simulink model "beta_estimators_simulink"  (R2017a)
settings: Solver=VariableStepAuto  StartTime=0.0  StopTime=10.0  FixedStep=1e-3  RelTol=1e-3
values from neighbouring files (symbols this model uses):
  Den_PDa = [1,(Na*Tsa-2)/(Na*Tsa+2)]    [rosbag_reader_simulink_GammaEstimators.m]
  FilterDTF = c2d(FilterCTF,Ts_filter,'tustin')    [rosbag_reader_simulink_GammaEstimators.m]
  Kp = 10*2*pi    (= 62.8318530718)    [rosbag_reader_simulink_GammaEstimators.m]    (also in taraPDscript.m = 628.318530718)
  Num_PDa = [(Kpa*(2+Na*Tsa)+2*Kda*Na)/(2+Na*Tsa),(-2*Kpa+Na*Tsa*Kpa-2*Kda*Na)/(2+Na*Tsa)]    [rosbag_reader_simulink_GammaEstimators.m]
  x0_acc = [X_opt.Data(1),Y_opt.Data(1),gamma_opt_spline.Data(1),V_opt.Data(1)]    [rosbag_reader_simulink_GammaEstimators.m]
  x0_vel = [X_opt.Data(1),Y_opt.Data(1),gamma_opt_spline.Data(1)]    [rosbag_reader_simulink_GammaEstimators.m]
undefined symbols (not defined in the file or in its folder): DiscIntNeverNeededParam
libraries: dspsigops x2
settings Model: Creator=bascetta  LastModifiedBy=marco
settings OptimizationCC: DefaultParameterBehavior=Inlined  PassReuseOutputArgsAs=Individual arguments  MaxStackSize=64
settings DebuggingCC: ParameterTunabilityLossMsg=error
settings HardwareCC: ProdBitPerPointer=32  ProdBitPerSizeT=32  ProdBitPerPtrDiffT=32  ProdLargestAtomicFloat=None  ProdIntDivRoundTo=Undefined  ProdEndianess=Unspecified  ProdWordSize=32  ProdHWDeviceType=Generic->Unspecified (assume 32-bit Generic)
settings SFSimCC: MATLABDynamicMemAlloc=off
settings RTWCC: SystemTargetFile=ert.tlc  TemplateMakefile=ert_default_tmf  Description=Embedded Coder  GenerateReport=on  Toolchain=Catkin  IncludeHyperlinkInReport=on  LaunchReport=on  GenerateTraceInfo=on  GenerateTraceReport=on  GenerateTraceReportSl=on  GenerateTraceReportSf=on  GenerateTraceReportEml=on
settings CodeAppCC: ForceParamTrailComments=on  IgnoreCustomStorageClasses=off  OperatorAnnotations=on  SimulinkDataObjDesc=on  SFDataObjDesc=on  MATLABFcnDesc=on  InsertBlockDesc=on  MATLABSourceComments=on
settings ERTTargetCC: ERTCustomFileTemplate=example_file_process.tlc

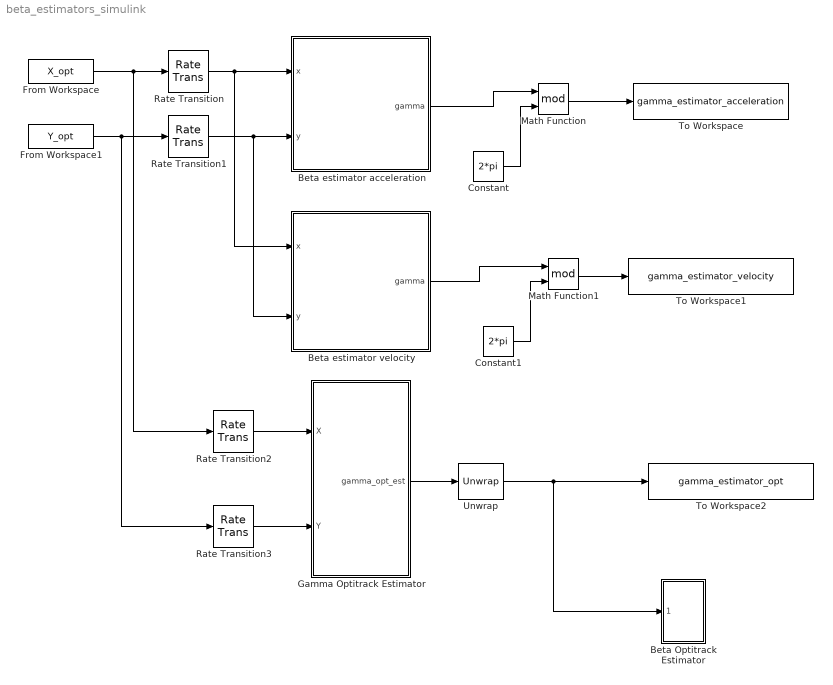
== system beta_estimators_simulink ==
  Beta Optitrack Estimator : Subsystem
  Beta estimator acceleration : Subsystem  TreatAsAtomicUnit=on  SystemSampleTime=1e-3
  Beta estimator velocity : Subsystem
  Constant : Constant  Value=2*pi
  Constant1 : Constant  Value=2*pi
  From Workspace : FromWorkspace  VariableName=X_opt  SampleTime=0  Interpolate=off  OutputAfterFinalValue=Holding final value
  From Workspace1 : FromWorkspace  VariableName=Y_opt  SampleTime=0  Interpolate=off  OutputAfterFinalValue=Holding final value
  Gamma Optitrack Estimator : Subsystem  TreatAsAtomicUnit=on  SystemSampleTime=0.01
  Math Function : Math  Operator=mod  OutputSignalType=real  SaturateOnIntegerOverflow=on
  Math Function1 : Math  Operator=mod  OutputSignalType=real  SaturateOnIntegerOverflow=on
  Rate Transition{,1..3} (4 alike) : RateTransition
  To Workspace : ToWorkspace  VariableName=gamma_estimator_acceleration  SaveFormat=Timeseries  SampleTime=-1
  To Workspace1 : ToWorkspace  VariableName=gamma_estimator_velocity  SaveFormat=Timeseries  SampleTime=-1
  To Workspace2 : ToWorkspace  VariableName=gamma_estimator_opt  SaveFormat=Timeseries  SampleTime=-1
  Unwrap : dspsigops/Unwrap  tol=pi  InputProcessing=Columns as channels (frame based)  running=off
  wires:
  From Workspace1/1 -> Rate Transition3/1, Rate Transition1/1
  Math Function/1 -> To Workspace/1
  Constant/1 -> Math Function/2
  Beta estimator acceleration/1(gamma) -> Math Function/1
  From Workspace/1 -> Rate Transition2/1, Rate Transition/1
  Math Function1/1 -> To Workspace1/1
  Constant1/1 -> Math Function1/2
  Beta estimator velocity/1(gamma) -> Math Function1/1
  Rate Transition/1 -> Beta estimator velocity/1(x), Beta estimator acceleration/1(x)
  Rate Transition1/1 -> Beta estimator velocity/2(y), Beta estimator acceleration/2(y)
  Rate Transition2/1 -> Gamma Optitrack Estimator/1(X)
  Rate Transition3/1 -> Gamma Optitrack Estimator/2(Y)
  Gamma Optitrack Estimator/1(gamma_opt_est) -> Unwrap/1
  Unwrap/1 -> Beta Optitrack Estimator/1(gamma_opt), To Workspace2/1

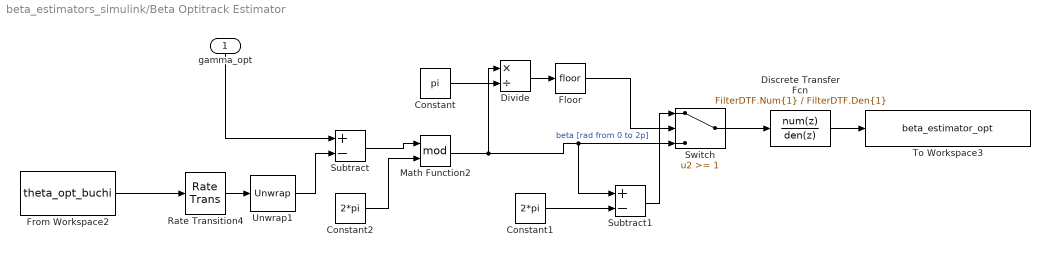
== system beta_estimators_simulink/Beta Optitrack Estimator ==
  gamma_opt : Inport
  Constant : Constant  Value=pi
  Constant1 : Constant  Value=2*pi
  Constant2 : Constant  Value=2*pi
  Discrete Transfer Fcn : DiscreteTransferFcn  Numerator=FilterDTF.Num{1}  Denominator=FilterDTF.Den{1}
  Divide : Product  Inputs=*/
  Floor : Rounding
  From Workspace2 : FromWorkspace  VariableName=theta_opt_buchi  SampleTime=0  Interpolate=off  OutputAfterFinalValue=Holding final value
  Math Function2 : Math  Operator=mod  SaturateOnIntegerOverflow=on
  Rate Transition4 : RateTransition  OutPortSampleTime=0.01
  Subtract : Sum  Inputs=+-
  Subtract1 : Sum  Inputs=+-
  Switch : Switch  Threshold=1
  To Workspace3 : ToWorkspace  VariableName=beta_estimator_opt  SaveFormat=Timeseries  SampleTime=-1
  Unwrap1 : dspsigops/Unwrap  tol=pi  InputProcessing=Columns as channels (frame based)  running=off
  wires:
  Rate Transition4/1 -> Unwrap1/1
  Subtract/1 -> Math Function2/1
  Unwrap1/1 -> Subtract/2
  Constant2/1 -> Math Function2/2
  gamma_opt/1 -> Subtract/1
  From Workspace2/1 -> Rate Transition4/1
  Switch/1 -> Discrete Transfer Fcn/1
  Math Function2/1 -> Divide/1, Subtract1/1, Switch/3  "beta [rad from 0 to 2p]"
  Divide/1 -> Floor/1
  Constant/1 -> Divide/2
  Floor/1 -> Switch/2
  Constant1/1 -> Subtract1/2
  Subtract1/1 -> Switch/1
  Discrete Transfer Fcn/1 -> To Workspace3/1

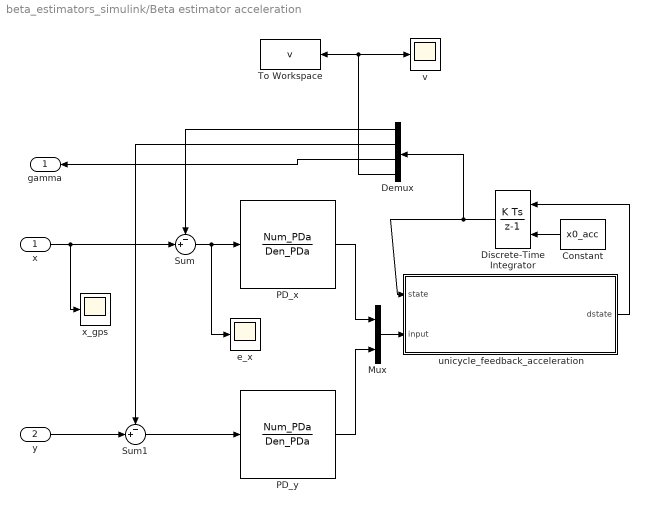
== system beta_estimators_simulink/Beta estimator acceleration ==
  x : Inport
  y : Inport  Port=2
  Constant : Constant  Value=x0_acc
  Demux : Demux
  Discrete-Time Integrator : DiscreteIntegrator  InitialConditionSource=external  InitialCondition=[0 0 0 0.1]  InitialConditionSetting=State (most efficient)  SampleTime=1e-3  ICPrevOutput=DiscIntNeverNeededParam  ICPrevScaledInput=DiscIntNeverNeededParam
  Mux : Mux  Inputs=2
  PD_x : DiscreteTransferFcn  Numerator=Num_PDa  Denominator=Den_PDa  SampleTime=0.001  a0EqualsOne=on
  PD_y : DiscreteTransferFcn  Numerator=Num_PDa  Denominator=Den_PDa  SampleTime=0.001  a0EqualsOne=on
  Sum : Sum  Inputs=-+|
  Sum1 : Sum  Inputs=-+|
  To Workspace : ToWorkspace  VariableName=v  SaveFormat=Timeseries  SampleTime=-1
  e_x : Scope
  unicycle_feedback_acceleration : MATLAB Function  TreatAsAtomicUnit=on
  v : Scope
  x_gps : Scope
  gamma : Outport
  wires:
  unicycle_feedback_acceleration/1(dstate) -> Discrete-Time Integrator/1
  Mux/1 -> unicycle_feedback_acceleration/2(input)
  Demux/1 -> Sum/1
  Sum/1 -> e_x/1, PD_x/1
  PD_x/1 -> Mux/1
  y/1 -> Sum1/2
  Demux/3 -> gamma/1
  Demux/2 -> Sum1/1
  Discrete-Time Integrator/1 -> unicycle_feedback_acceleration/1(state), Demux/1
  Demux/4 -> v/1, To Workspace/1
  x/1 -> x_gps/1, Sum/2
  Sum1/1 -> PD_y/1
  PD_y/1 -> Mux/2
  Constant/1 -> Discrete-Time Integrator/2

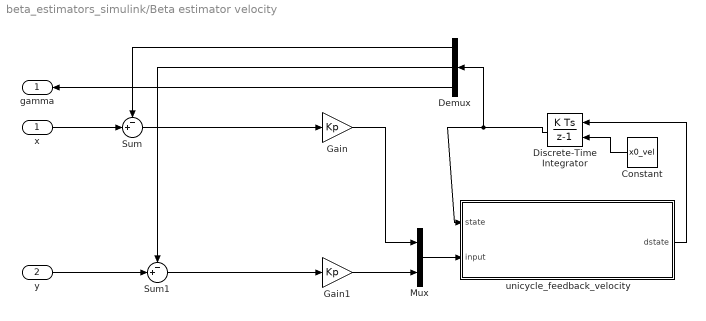
== system beta_estimators_simulink/Beta estimator velocity ==
  x : Inport
  y : Inport  Port=2
  Constant : Constant  Value=x0_vel
  Demux : Demux  Outputs=3
  Discrete-Time Integrator : DiscreteIntegrator  InitialConditionSource=external  InitialConditionSetting=State (most efficient)  SampleTime=0.001  ICPrevOutput=DiscIntNeverNeededParam  ICPrevScaledInput=DiscIntNeverNeededParam
  Gain : Gain  Gain=Kp
  Gain1 : Gain  Gain=Kp
  Mux : Mux  Inputs=2
  Sum : Sum  Inputs=-+|
  Sum1 : Sum  Inputs=-+|
  unicycle_feedback_velocity : MATLAB Function  TreatAsAtomicUnit=on
  gamma : Outport
  wires:
  Demux/3 -> gamma/1
  y/1 -> Sum1/2
  Demux/1 -> Sum/1
  Gain1/1 -> Mux/2
  Gain/1 -> Mux/1
  Mux/1 -> unicycle_feedback_velocity/2(input)
  Demux/2 -> Sum1/1
  x/1 -> Sum/2
  unicycle_feedback_velocity/1(dstate) -> Discrete-Time Integrator/1
  Discrete-Time Integrator/1 -> Demux/1, unicycle_feedback_velocity/1(state)
  Sum1/1 -> Gain1/1
  Sum/1 -> Gain/1
  Constant/1 -> Discrete-Time Integrator/2

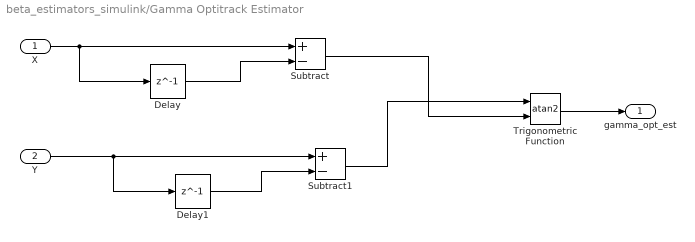
== system beta_estimators_simulink/Gamma Optitrack Estimator ==
  X : Inport
  Y : Inport  Port=2
  Delay : Delay  DelayLength=1  InitialCondition=0
  Delay1 : Delay  DelayLength=1  InitialCondition=0
  Subtract : Sum  Inputs=+-
  Subtract1 : Sum  Inputs=+-
  Trigonometric Function : Trigonometry  Operator=atan2
  gamma_opt_est : Outport
  wires:
  Trigonometric Function/1 -> gamma_opt_est/1
  X/1 -> Delay/1, Subtract/1
  Delay/1 -> Subtract/2
  Subtract/1 -> Trigonometric Function/2
  Subtract1/1 -> Trigonometric Function/1
  Delay1/1 -> Subtract1/2
  Y/1 -> Delay1/1, Subtract1/1

== matlab function beta_estimators_simulink/Beta estimator velocity/unicycle_feedback_velocity ==
  data: state input size=3; dstate output size=3; input input size=2; p parameter size=1
function dstate = unicycle_feedback_velocity(state,input,p)

% State and input variables
x     = state(1);
y     = state(2);
gamma = state(3); % theta+beta

vxp   = input(1);
vyp   = input(2);


% Model equations
dstate = zeros(3,1);
dstate(1) = vxp*cos(gamma)^2+vyp*sin(gamma)*cos(gamma);
dstate(2) = vxp*sin(gamma)*cos(gamma)+vyp*sin(gamma)^2;
dstate(3) = (vyp*cos(gamma)-vxp*sin(gamma))/p;

== matlab function beta_estimators_simulink/Beta estimator acceleration/unicycle_feedback_acceleration ==
  data: state input size=4; dstate output size=4; input input size=2
function dstate = unicycle_feedback_acceleration(state,input)

% State and input variables
x     = state(1); %[m]
y     = state(2); %[m]
gamma = state(3); % theta+beta [rad]
v     = state(4); %[m/s]

ax    = input(1); %[m/s^2]
ay    = input(2); %[m/s^2]

    % Model equations
    dstate = zeros(4,1);
    dstate(1) = v*cos(gamma); %dx/dt
    dstate(2) = v*sin(gamma); %dy/dt
    dstate(3) = (ay*cos(gamma)-ax*sin(gamma))/v; %d(gamma)/dt
    dstate(4) = ax*cos(gamma)+ay*sin(gamma); %dv/dt
end
